simulink model "ADC_Controller_Trajectory_Tracking_Turb"  (R2017b)
settings: Solver=VariableStepAuto  StartTime=0.0  StopTime=200  FixedStep=0.01  RelTol=1e-3
values from neighbouring files (symbols this model uses):
  A_define = A(1:12,1:12)    [F16_init.m]
  A_la_define = A_define([2,4,6,9,10,12],[2,4,6,9,10,12])    [Controller_para.m]
  A_lon_define = A_define([1,3,5,7,8,11],[1,3,5,7,8,11])    [Controller_para.m]
  airSpeed = 393.720000000000    (= 393.72)    [F16_init.m]
  alpha0 = trimAlpha*180/pi    (= 6.62393794015)    [F16_init.m]
  altitude = 9843    [F16_init.m]
  B_define = A(1:12,13:16)    [F16_init.m]
  B_la_define = B_define([2,4,6,9,10,12],3:4)    [Controller_para.m]
  B_lon_define = B_define([1,3,5,7,8,11],1:2)    [Controller_para.m]
  b_ref = 30.0    (= 30)    [F16_init.m]
  C_la = [1,0,zeros(1,4)]    [F16_init.m]
  C_lon = [1,0,zeros(1,4);0,1,zeros(1,4)]    [F16_init.m]
  CC_la = P_la * B_la_define    [Controller_para.m]
  CC_lon = P_lon * B_lon_define    [Controller_para.m]
  dLEF = 0    [F16_init.m]
  fi_flag = 1    [F16_init.m]
  Ki_la = -k_la(:,9)    [F16_init.m]
  Ki_lon = -k_lon(:,9:10)    [F16_init.m]
  kp_la = Kp_define(3:4,[2,4,6,9,10,12])    [Controller_para.m]    (also in F16_init.m)
  kp_lon = Kp_define(1:2,[1,3,5,7,8,11])    [Controller_para.m]    (also in F16_init.m)
  mass = 636.94    [F16_init.m]
  trim_ail = 0.00874607850103852    (= 0.00874607850104)    [F16_init.m]
  trim_control = [trim_thrust;trim_ele;trim_ail;trim_rud]    [F16_init.m]
  trim_ele = -2.97973164860638    (= -2.97973164861)    [F16_init.m]
  trim_rud = 0.0680302158182712    (= 0.0680302158183)    [F16_init.m]
  trim_state = [0;0;0;0;trimAlpha;0;airSpeed;trimAlpha;0;0;0;0]    [F16_init.m]
  trim_thrust = 2279.08519954656    (= 2279.08519955)    [F16_init.m]
undefined symbols (not defined in the file or in its folder): F, MIL
libraries: aerolibconvert2 x7, aerolibasang x4, aerolibobsolete x2, aerolibwind2 x1, aerolibatmos2 x1, aerolibadyn x1
settings Model: Creator=Ma  LastModifiedBy=Jinrui
settings CodeAppCC: StateflowObjectComments=on

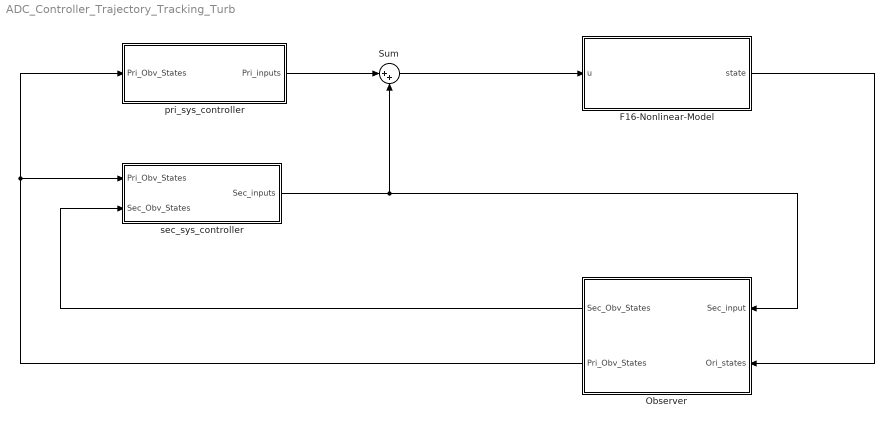
== system ADC_Controller_Trajectory_Tracking_Turb ==
  F16-Nonlinear-Model : Subsystem
  Observer : Subsystem
  Sum : Sum  Inputs=|++
  pri_sys_controller : Subsystem
  sec_sys_controller : Subsystem
  wires:
  pri_sys_controller/1(Pri_inputs) -> Sum/1
  Sum/1 -> F16-Nonlinear-Model/1(u)
  Observer/2(Pri_Obv_States) -> sec_sys_controller/1(Pri_Obv_States), pri_sys_controller/1(Pri_Obv_States)
  Observer/1(Sec_Obv_States) -> sec_sys_controller/2(Sec_Obv_States)
  F16-Nonlinear-Model/1(state) -> Observer/2(Ori_states)
  sec_sys_controller/1(Sec_inputs) -> Sum/2, Observer/1(Sec_input)

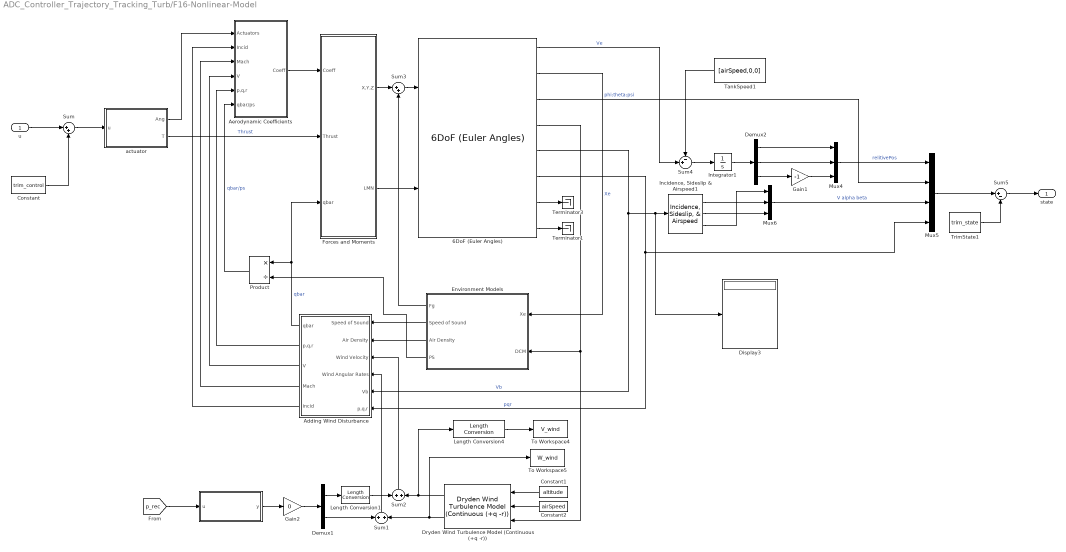
== system ADC_Controller_Trajectory_Tracking_Turb/F16-Nonlinear-Model ==
  u : Inport
  " " : MATLAB Function  TreatAsAtomicUnit=on
  6DoF (Euler Angles) : aerolibobsolete/6DoF (Euler Angles)  units=English (Velocity in ft/s)  mtype=Fixed  rep=Euler Angles  xme_0=xme_0  Vm_0=Vmw  eul_0=Euler_0  pm_0=pm_0  mass_0=mass  mass_e=0.5  mass_f=2.0  inertia=Inertia  inertia_e=eye(3)  inertia_f=2*eye(3)  k_quat=1.0
      settings: SourceProductName=Aerospace Blockset  SourceProductBaseCode=AE
  Adding Wind Disturbance : Subsystem
  Aerodynamic Coefficients : Subsystem
  Constant : Constant  Value=trim_control
  Constant1 : Constant  Value=altitude
  Constant2 : Constant  Value=airSpeed
  Demux1 : Demux  Outputs=2
  Demux2 : Demux  Outputs=3
  Display3 : Display
  Dryden Wind Turbulence Model (Continuous (+q -r)) : aerolibwind2/Dryden Wind Turbulence Model  (Continuous (+q -r))  units=English (Velocity in ft/s)  spec=MIL-F-8785C  model=Continuous Dryden (+q -r)  W20=15  Wdeg=0  TurbProb=10^-1  L_high=533.4  Wingspan=10  ts=0.1  Seed=1+fix(3650*rand(1,4))  T_on=on
      settings: SourceProductName=Aerospace Blockset
  Environment Models : Subsystem
  Forces and Moments : Subsystem
  Gain1 : Gain  Gain=-1
  Gain2 : Gain  Gain=0
  "Incidence, Sideslip & Airspeed1" : aerolibasang/Incidence, Sideslip, & Airspeed
      settings: SourceProductName=Aerospace Blockset
  Integrator1 : Integrator
  Length Conversion1 : aerolibconvert2/Length Conversion  IU=m  OU=ft
  Length Conversion4 : aerolibconvert2/Length Conversion  IU=ft  OU=m
  Mux4 : Mux  Inputs=3
  Mux5 : Mux
  Mux6 : Mux  Inputs=3
  Product : Product  Inputs=*/  SaturateOnIntegerOverflow=on  InputSameDT=on  OutDataTypeStr=Inherit: Same as first input
  Sum : Sum  Inputs=|++
  Sum1 : Sum  Inputs=+|+
  Sum2 : Sum  Inputs=+|+
  Sum3 : Sum  Inputs=|++  SaturateOnIntegerOverflow=on  InputSameDT=on  OutDataTypeStr=Inherit: Same as first input
  Sum4 : Sum  Inputs=-+|
  Sum5 : Sum  Inputs=|+-
  TankSpeed1 : Constant  Value=[airSpeed,0,0]
  Terminator1 : Terminator
  Terminator3 : Terminator
  To Workspace4 : ToWorkspace  VariableName=V_wind  SaveFormat=Structure With Time  SampleTime=-1
  To Workspace5 : ToWorkspace  VariableName=W_wind  SaveFormat=Structure With Time  SampleTime=-1
  TrimState1 : Constant  Value=trim_state
  actuator : Subsystem
  state : Outport
  wires:
  6DoF (Euler Angles)/8 -> Terminator1/1
  6DoF (Euler Angles)/7 -> Terminator3/1
  6DoF (Euler Angles)/4 -> Dryden Wind Turbulence Model (Continuous (+q -r))/3, Environment Models/2(DCM)
  Adding Wind Disturbance/5(Incid) -> Aerodynamic Coefficients/2(Incid)
  Aerodynamic Coefficients/1(Coeff) -> Forces and Moments/1(Coeff)
  Environment Models/2(Speed of Sound) -> Adding Wind Disturbance/1(Speed of Sound)
  Environment Models/3(Air Density) -> Adding Wind Disturbance/2(Air Density)
  Forces and Moments/2(LMN) -> 6DoF (Euler Angles)/2
  Adding Wind Disturbance/1(qbar) -> Forces and Moments/3(qbar), Product/1  "qbar"
  Forces and Moments/1(X,Y,Z) -> Sum3/1
  Sum3/1 -> 6DoF (Euler Angles)/1
  Environment Models/1(Fg) -> Sum3/2
  Adding Wind Disturbance/3(V) -> Aerodynamic Coefficients/4(V)
  Adding Wind Disturbance/4(Mach) -> Aerodynamic Coefficients/3(Mach)
  Adding Wind Disturbance/2("p,q,r ") -> Aerodynamic Coefficients/5(p,q,r)
  Environment Models/4(PS) -> Product/2
  Product/1 -> Aerodynamic Coefficients/6(qbar/ps)  "qbar/ps"
  actuator/2(T) -> Forces and Moments/2(Thrust)  "Thrust"
  actuator/1(Ang) -> Aerodynamic Coefficients/1(Actuators)
  6DoF (Euler Angles)/3 -> Mux5/2  "phi;theta;psi"
  "Incidence, Sideslip & Airspeed1"/1 -> Mux6/2
  "Incidence, Sideslip & Airspeed1"/2 -> Mux6/3
  Mux6/1 -> Mux5/3  "V alpha beta"
  6DoF (Euler Angles)/6 -> Adding Wind Disturbance/6(p,q,r), Mux5/4  "pqr"
  6DoF (Euler Angles)/5 -> Adding Wind Disturbance/5(Vb), Display3/1, "Incidence, Sideslip & Airspeed1"/1  "Vb"
  Mux5/1 -> Sum5/1
  TrimState1/1 -> Sum5/2
  Sum5/1 -> state/1
  Demux2/2 -> Mux4/2
  Demux2/3 -> Gain1/1
  Mux4/1 -> Mux5/1  "relitivePos"
  Demux2/1 -> Mux4/1
  Gain1/1 -> Mux4/3
  Sum4/1 -> Integrator1/1
  Integrator1/1 -> Demux2/1
  6DoF (Euler Angles)/2 -> Environment Models/1(Xe)  "Xe"
  6DoF (Euler Angles)/1 -> Sum4/2  "Ve"
  TankSpeed1/1 -> Sum4/1
  "Incidence, Sideslip & Airspeed1"/3 -> Mux6/1
  Sum/1 -> actuator/1(u)
  Constant/1 -> Sum/2
  u/1 -> Sum/1
  Constant1/1 -> Dryden Wind Turbulence Model (Continuous (+q -r))/1
  Constant2/1 -> Dryden Wind Turbulence Model (Continuous (+q -r))/2
  [p_rec] -> " "/1(u)
  " "/1(y) -> Gain2/1
  Demux1/2 -> Sum1/1
  Sum1/1 -> Adding Wind Disturbance/4(Wind Angular Rates)
  Dryden Wind Turbulence Model (Continuous (+q -r))/1 -> Length Conversion4/1, Sum2/2
  Demux1/1 -> Length Conversion1/1
  Sum2/1 -> Adding Wind Disturbance/3(Wind Velocity)
  Gain2/1 -> Demux1/1
  Length Conversion4/1 -> To Workspace4/1
  Dryden Wind Turbulence Model (Continuous (+q -r))/2 -> To Workspace5/1, Sum1/2
  Length Conversion1/1 -> Sum2/1

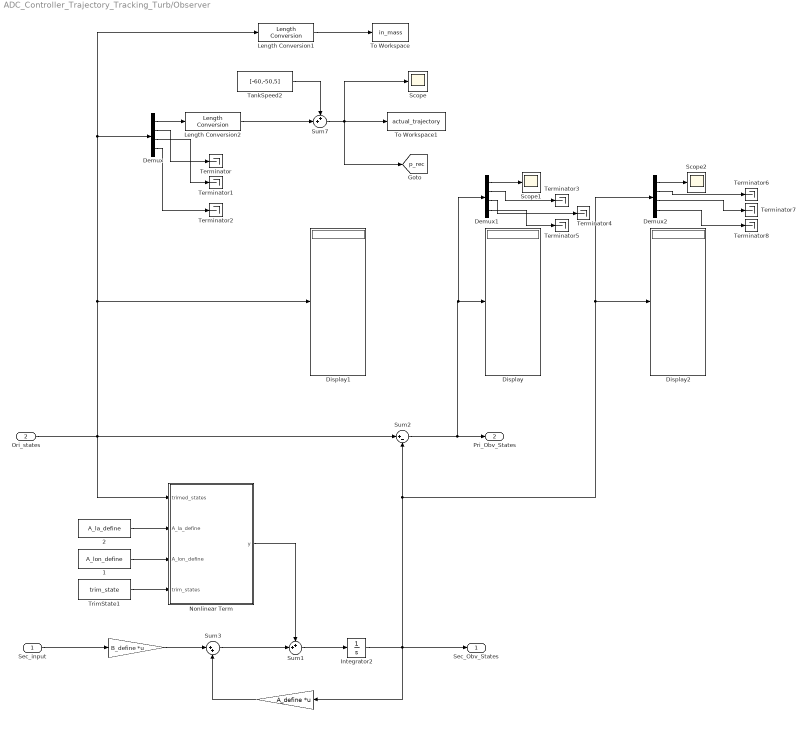
== system ADC_Controller_Trajectory_Tracking_Turb/Observer ==
  Sec_input : Inport
  Ori_states : Inport  Port=2
  " " : Gain  Gain=A_define  Multiplication=Matrix(K*u) (u vector)
  "  " : Gain  Gain=B_define  Multiplication=Matrix(K*u) (u vector)
  " 1" : Constant  Value=A_lon_define
  " 2" : Constant  Value=A_la_define
  Demux : Demux
  Demux1 : Demux
  Demux2 : Demux
  Display : Display
  Display1 : Display
  Display2 : Display
  Integrator2 : Integrator  InitialCondition=zeros(12,1)
  Length Conversion1 : aerolibconvert2/Length Conversion  IU=ft  OU=m
  Length Conversion2 : aerolibconvert2/Length Conversion  IU=ft  OU=m
  Nonlinear Term : MATLAB Function  TreatAsAtomicUnit=on
  Scope : Scope
  Scope1 : Scope
  Scope2 : Scope
  Sum1 : Sum  Inputs=++|
  Sum2 : Sum  Inputs=|+-
  Sum3 : Sum  Inputs=|++
  Sum7 : Sum  Inputs=++|
  TankSpeed2 : Constant  Value=[-60,-50,5]
  Terminator{,1..8} (9 alike) : Terminator
  To Workspace : ToWorkspace  VariableName=in_mass  SaveFormat=Structure With Time  SampleTime=-1
  To Workspace1 : ToWorkspace  VariableName=actual_trajectory  SaveFormat=Structure With Time  SampleTime=-1
  TrimState1 : Constant  Value=trim_state
  Sec_Obv_States : Outport
  Pri_Obv_States : Outport  Port=2
  tag scope: p_rec=global
  wires:
  Sec_input/1 -> "  "/1
  "  "/1 -> Sum3/1
  " "/1 -> Sum3/2
  Sum3/1 -> Sum1/2
  Sum1/1 -> Integrator2/1
  Integrator2/1 -> Sec_Obv_States/1, " "/1, Demux2/1, Display2/1, Sum2/2
  Sum2/1 -> Demux1/1, Display/1, Pri_Obv_States/1
  " 1"/1 -> Nonlinear Term/3(A_lon_define)
  " 2"/1 -> Nonlinear Term/2(A_la_define)
  Demux/1 -> Length Conversion2/1
  Demux1/1 -> Scope1/1
  Demux2/1 -> Scope2/1
  Nonlinear Term/1(y) -> Sum1/1
  TrimState1/1 -> Nonlinear Term/4(trim_states)
  Length Conversion1/1 -> To Workspace/1
  Ori_states/1 -> Sum2/1, Display1/1, Demux/1, Length Conversion1/1, Nonlinear Term/1(trimed_states)
  Length Conversion2/1 -> Sum7/2
  Sum7/1 -> Scope/1, To Workspace1/1, [p_rec]
  TankSpeed2/1 -> Sum7/1
  Demux/2 -> Terminator/1
  Demux/3 -> Terminator1/1
  Demux/4 -> Terminator2/1
  Demux1/2 -> Terminator3/1
  Demux1/3 -> Terminator4/1
  Demux1/4 -> Terminator5/1
  Demux2/4 -> Terminator8/1
  Demux2/3 -> Terminator7/1
  Demux2/2 -> Terminator6/1

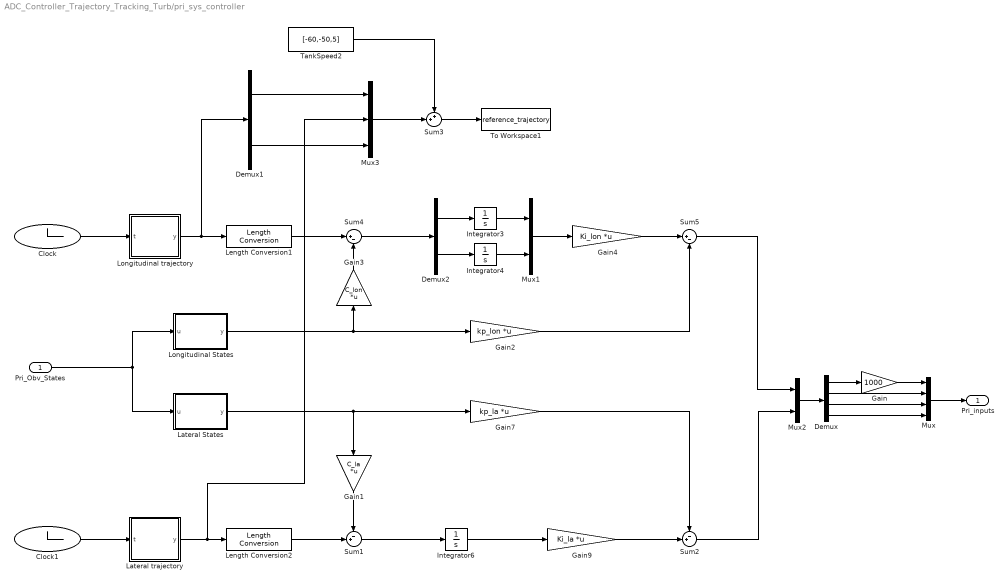
== system ADC_Controller_Trajectory_Tracking_Turb/pri_sys_controller ==
  Pri_Obv_States : Inport
  Clock : Clock
      settings: Decimation=50
  Clock1 : Clock
      settings: Decimation=50
  Demux : Demux
  Demux1 : Demux  Outputs=2
  Demux2 : Demux  Outputs=2
  Gain : Gain  Gain=1000
  Gain1 : Gain  Gain=C_la  Multiplication=Matrix(K*u) (u vector)
  Gain2 : Gain  Gain=kp_lon  Multiplication=Matrix(K*u) (u vector)
  Gain3 : Gain  Gain=C_lon  Multiplication=Matrix(K*u) (u vector)
  Gain4 : Gain  Gain=Ki_lon  Multiplication=Matrix(K*u) (u vector)
  Gain7 : Gain  Gain=kp_la  Multiplication=Matrix(K*u) (u vector)
  Gain9 : Gain  Gain=Ki_la  Multiplication=Matrix(K*u) (u vector)
  Integrator3 : Integrator
  Integrator4 : Integrator
  Integrator6 : Integrator
  Lateral States : MATLAB Function  TreatAsAtomicUnit=on
  Lateral trajectory : MATLAB Function  TreatAsAtomicUnit=on
  Length Conversion1 : aerolibconvert2/Length Conversion  IU=m  OU=ft
  Length Conversion2 : aerolibconvert2/Length Conversion  IU=m  OU=ft
  Longitudinal States : MATLAB Function  TreatAsAtomicUnit=on
  Longitudinal trajectory : MATLAB Function  TreatAsAtomicUnit=on
  Mux : Mux
  Mux1 : Mux  Inputs=2
  Mux2 : Mux  Inputs=2
  Mux3 : Mux  Inputs=3
  Sum1 : Sum  Inputs=-+|
  Sum2 : Sum  Inputs=-+|
  Sum3 : Sum  Inputs=++|
  Sum4 : Sum  Inputs=|+-
  Sum5 : Sum  Inputs=|+-
  TankSpeed2 : Constant  Value=[-60,-50,5]
  To Workspace1 : ToWorkspace  VariableName=reference_trajectory  SaveFormat=Structure With Time  SampleTime=-1
  Pri_inputs : Outport
  wires:
  Pri_Obv_States/1 -> Longitudinal States/1(u), Lateral States/1(u)
  Gain2/1 -> Sum5/2
  Longitudinal trajectory/1(y) -> Demux1/1, Length Conversion1/1
  Sum4/1 -> Demux2/1
  Demux2/2 -> Integrator4/1
  Integrator4/1 -> Mux1/2
  Integrator3/1 -> Mux1/1
  Mux1/1 -> Gain4/1
  Gain3/1 -> Sum4/2
  Gain4/1 -> Sum5/1
  Clock/1 -> Longitudinal trajectory/1(t)
  Length Conversion1/1 -> Sum4/1
  Demux/2 -> Mux/2
  Demux/3 -> Mux/3
  Demux/4 -> Mux/4
  Demux/1 -> Gain/1
  Gain/1 -> Mux/1
  Mux/1 -> Pri_inputs/1
  Lateral trajectory/1(y) -> Mux3/2, Length Conversion2/1
  Sum1/1 -> Integrator6/1
  Integrator6/1 -> Gain9/1
  Clock1/1 -> Lateral trajectory/1(t)
  Longitudinal States/1(y) -> Gain2/1, Gain3/1
  Lateral States/1(y) -> Gain7/1, Gain1/1
  Length Conversion2/1 -> Sum1/2
  Gain1/1 -> Sum1/1
  Gain9/1 -> Sum2/2
  Gain7/1 -> Sum2/1
  Sum5/1 -> Mux2/1
  Sum2/1 -> Mux2/2
  Demux2/1 -> Integrator3/1
  Mux2/1 -> Demux/1
  Demux1/1 -> Mux3/1
  Demux1/2 -> Mux3/3
  Sum3/1 -> To Workspace1/1
  Mux3/1 -> Sum3/2
  TankSpeed2/1 -> Sum3/1

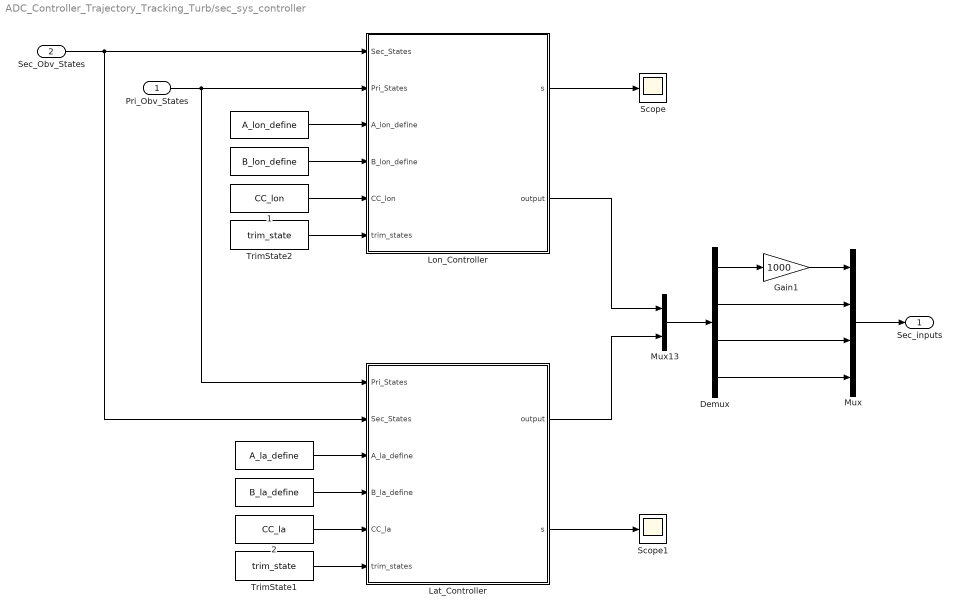
== system ADC_Controller_Trajectory_Tracking_Turb/sec_sys_controller ==
  Pri_Obv_States : Inport
  Sec_Obv_States : Inport  Port=2
  " " : Constant  Value=A_lon_define
  "    " : Constant  Value=B_lon_define
  "     " : Constant  Value=A_la_define
  "      " : Constant  Value=B_la_define
  "    1" : Constant  Value=CC_lon
  "    2" : Constant  Value=CC_la
  Demux : Demux
  Gain1 : Gain  Gain=1000
  Lat_Controller : MATLAB Function  TreatAsAtomicUnit=on
  Lon_Controller : MATLAB Function  TreatAsAtomicUnit=on
  Mux : Mux
  Mux13 : Mux  Inputs=2
  Scope : Scope
  Scope1 : Scope
  TrimState1 : Constant  Value=trim_state
  TrimState2 : Constant  Value=trim_state
  Sec_inputs : Outport
  wires:
  Demux/1 -> Gain1/1
  Gain1/1 -> Mux/1
  Mux/1 -> Sec_inputs/1
  Demux/2 -> Mux/2
  Demux/3 -> Mux/3
  Demux/4 -> Mux/4
  Lon_Controller/2(output) -> Mux13/1
  " "/1 -> Lon_Controller/3(A_lon_define)
  "    "/1 -> Lon_Controller/4(B_lon_define)
  "     "/1 -> Lat_Controller/3(A_la_define)
  "      "/1 -> Lat_Controller/4(B_la_define)
  Lat_Controller/1(output) -> Mux13/2
  "    1"/1 -> Lon_Controller/5(CC_lon)
  "    2"/1 -> Lat_Controller/5(CC_la)
  Lon_Controller/1(s) -> Scope/1
  Lat_Controller/2(s) -> Scope1/1
  Mux13/1 -> Demux/1
  Sec_Obv_States/1 -> Lat_Controller/2(Sec_States), Lon_Controller/1(Sec_States)
  Pri_Obv_States/1 -> Lat_Controller/1(Pri_States), Lon_Controller/2(Pri_States)
  TrimState1/1 -> Lat_Controller/6(trim_states)
  TrimState2/1 -> Lon_Controller/6(trim_states)

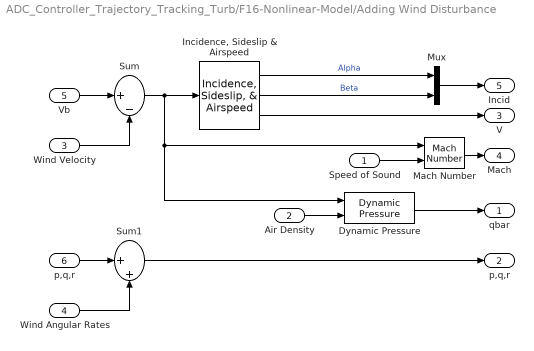
== system ADC_Controller_Trajectory_Tracking_Turb/F16-Nonlinear-Model/Adding Wind Disturbance ==
  Speed of Sound : Inport
  Air Density : Inport  Port=2
  Wind Velocity : Inport  Port=3  PortDimensions=3
  Wind Angular Rates : Inport  Port=4  PortDimensions=3
  Vb : Inport  Port=5  PortDimensions=3
  p,q,r : Inport  Port=6  PortDimensions=3
  Dynamic Pressure : aerolibasang/Dynamic Pressure
  "Incidence, Sideslip & Airspeed" : aerolibasang/Incidence, Sideslip, & Airspeed
      settings: SourceProductName=Aerospace Blockset
  Mach Number : aerolibasang/Mach Number
      settings: SourceProductName=Aerospace Blockset  SourceProductBaseCode=AE
  Mux : Mux  Inputs=2
  Sum : Sum  Inputs=|+-  SaturateOnIntegerOverflow=on  InputSameDT=on  OutDataTypeStr=Inherit: Same as first input
  Sum1 : Sum  Inputs=|++  SaturateOnIntegerOverflow=on  InputSameDT=on  OutDataTypeStr=Inherit: Same as first input
  qbar : Outport  InitialOutput=0
  "p,q,r " : Outport  Port=2
  V : Outport  Port=3
  Mach : Outport  Port=4
  Incid : Outport  Port=5
  wires:
  "Incidence, Sideslip & Airspeed"/3 -> V/1
  Dynamic Pressure/1 -> qbar/1
  Air Density/1 -> Dynamic Pressure/2
  Mach Number/1 -> Mach/1
  Sum/1 -> Dynamic Pressure/1, Mach Number/1, "Incidence, Sideslip & Airspeed"/1
  Vb/1 -> Sum/1
  Speed of Sound/1 -> Mach Number/2
  Wind Velocity/1 -> Sum/2
  "Incidence, Sideslip & Airspeed"/2 -> Mux/2  "Beta"
  Mux/1 -> Incid/1
  "Incidence, Sideslip & Airspeed"/1 -> Mux/1  "Alpha"
  p,q,r/1 -> Sum1/1
  Wind Angular Rates/1 -> Sum1/2
  Sum1/1 -> "p,q,r "/1

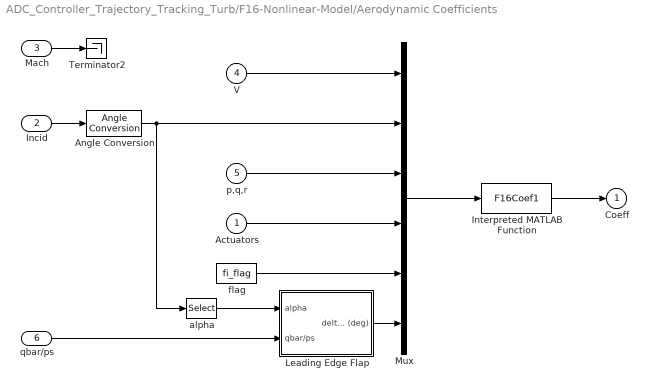
== system ADC_Controller_Trajectory_Tracking_Turb/F16-Nonlinear-Model/Aerodynamic Coefficients ==
  Actuators : Inport
  Incid : Inport  Port=2
  Mach : Inport  Port=3
  V : Inport  Port=4
  p,q,r : Inport  Port=5
  qbar/ps : Inport  Port=6
  Angle Conversion : aerolibconvert2/Angle Conversion  IU=rad  OU=deg
  Interpreted MATLAB Function : MATLABFcn  MATLABFcn=F16Coef1  OutputDimensions=6
  Leading Edge Flap : Subsystem
  Mux : Mux  Inputs=6
  Terminator2 : Terminator
  alpha : Selector  InputPortWidth=2  IndexOptions=Index vector (dialog)  Indices=1  OutputSizes=1
  flag : Constant  Value=fi_flag
  Coeff : Outport  InitialOutput=0
  wires:
  Angle Conversion/1 -> alpha/1, Mux/2
  Incid/1 -> Angle Conversion/1
  qbar/ps/1 -> Leading Edge Flap/2(qbar/ps)
  alpha/1 -> Leading Edge Flap/1(alpha)
  V/1 -> Mux/1
  p,q,r/1 -> Mux/3
  Actuators/1 -> Mux/4
  flag/1 -> Mux/5
  Mach/1 -> Terminator2/1
  Interpreted MATLAB Function/1 -> Coeff/1
  Mux/1 -> Interpreted MATLAB Function/1
  Leading Edge Flap/1(delta_lef (deg)) -> Mux/6

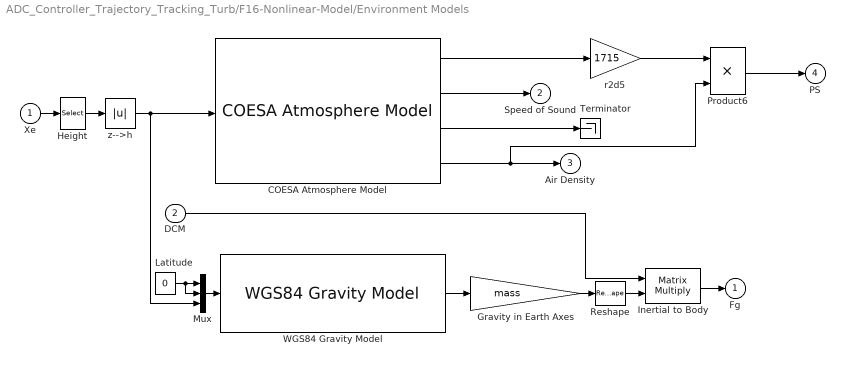
== system ADC_Controller_Trajectory_Tracking_Turb/F16-Nonlinear-Model/Environment Models ==
  Xe : Inport  PortDimensions=3
  DCM : Inport  Port=2
  COESA Atmosphere Model : aerolibatmos2/COESA Atmosphere Model  units=English (Velocity in ft/s)  spec=1976 COESA-extended U.S. Standard Atmosphere  model=Profile  profile_var=High temperature  profile_percent=10%  profile_alt=5 km (16404 ft)  envelope_var=High temperature  envelope_percent=1%  action=None
  Gravity in Earth Axes : Gain  Gain=mass  SaturateOnIntegerOverflow=on  OutDataTypeStr=Inherit: Same as input  ParamDataTypeStr=Inherit: Same as input
  Height : Selector  InputPortWidth=3  IndexOptions=Index vector (dialog)  Indices=[3]  OutputSizes=1
  Inertial to Body : Product  Multiplication=Matrix(*)  SaturateOnIntegerOverflow=on  InputSameDT=on  OutDataTypeStr=Inherit: Same as first input
  Latitude : Constant  Value=0
  Mux : Mux  Inputs=3
  Product6 : Product  Inputs=**  SaturateOnIntegerOverflow=on  InputSameDT=on  OutDataTypeStr=Inherit: Same as first input
  Reshape : Reshape
  Terminator : Terminator
  "WGS84 Gravity Model " : aerolibobsolete/WGS84 Gravity Model   model=WGS84 Taylor Series  units=English  no_atmos=on  precessing=on  jd_loc=off  month=October  day=10  year=2004  no_centrifugal=on  action=None
      settings: SourceProductName=Aerospace Blockset  SourceProductBaseCode=AE
  r2d5 : Gain  Gain=1715  SaturateOnIntegerOverflow=on  OutDataTypeStr=Inherit: Same as input  ParamDataTypeStr=Inherit: Same as input
  z-->h : Abs  SaturateOnIntegerOverflow=on
  Fg : Outport  InitialOutput=0
  Speed of Sound : Outport  Port=2  InitialOutput=0
  Air Density : Outport  Port=3  InitialOutput=0
  PS : Outport  Port=4
  wires:
  Reshape/1 -> Inertial to Body/2
  Mux/1 -> "WGS84 Gravity Model "/1
  z-->h/1 -> Mux/3, COESA Atmosphere Model/1
  COESA Atmosphere Model/2 -> Speed of Sound/1
  COESA Atmosphere Model/3 -> Terminator/1
  Height/1 -> z-->h/1
  Xe/1 -> Height/1
  Latitude/1 -> Mux/2, Mux/1
  "WGS84 Gravity Model "/1 -> Gravity in Earth Axes/1
  Gravity in Earth Axes/1 -> Reshape/1
  DCM/1 -> Inertial to Body/1
  Inertial to Body/1 -> Fg/1
  COESA Atmosphere Model/4 -> Product6/2, Air Density/1
  COESA Atmosphere Model/1 -> r2d5/1
  Product6/1 -> PS/1
  r2d5/1 -> Product6/1

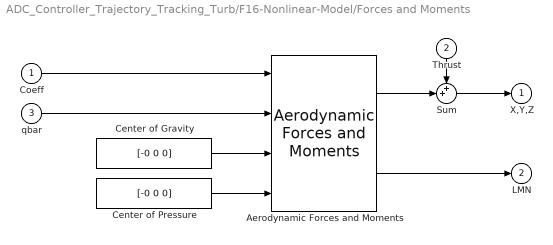
== system ADC_Controller_Trajectory_Tracking_Turb/F16-Nonlinear-Model/Forces and Moments ==
  Coeff : Inport
  Thrust : Inport  Port=2
  qbar : Inport  Port=3
  "Aerodynamic Forces and Moments " : aerolibadyn/Aerodynamic Forces and Moments   inputAxes=Body  outputForceAxes=Body  outputMomentAxes=Body  S=S_ref  b=b_ref  cbar=d_ref
      settings: SourceProductName=Aerospace Blockset
  Center of Gravity : Constant  Value=[-0 0 0]
  Center of Pressure : Constant  Value=[-0 0 0]
  Sum : Sum  Inputs=++|  SaturateOnIntegerOverflow=on  InputSameDT=on  OutDataTypeStr=Inherit: Same as first input
  X,Y,Z : Outport  InitialOutput=0
  LMN : Outport  Port=2  InitialOutput=0
  wires:
  Center of Pressure/1 -> "Aerodynamic Forces and Moments "/4
  Center of Gravity/1 -> "Aerodynamic Forces and Moments "/3
  "Aerodynamic Forces and Moments "/1 -> Sum/2
  "Aerodynamic Forces and Moments "/2 -> LMN/1
  Sum/1 -> X,Y,Z/1
  Thrust/1 -> Sum/1
  qbar/1 -> "Aerodynamic Forces and Moments "/2
  Coeff/1 -> "Aerodynamic Forces and Moments "/1

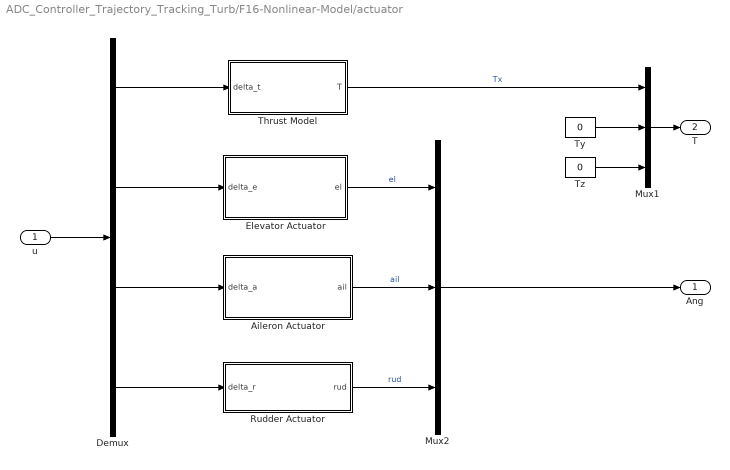
== system ADC_Controller_Trajectory_Tracking_Turb/F16-Nonlinear-Model/actuator ==
  u : Inport
  Aileron Actuator : Subsystem
  Demux : Demux
  Elevator Actuator : Subsystem
  Mux1 : Mux  Inputs=3
  Mux2 : Mux  Inputs=3
  Rudder Actuator : Subsystem
  Thrust Model : Subsystem
  Ty : Constant  Value=0
  Tz : Constant  Value=0
  Ang : Outport
  T : Outport  Port=2
  wires:
  u/1 -> Demux/1
  Mux2/1 -> Ang/1
  Thrust Model/1(T) -> Mux1/1  "Tx"
  Ty/1 -> Mux1/2
  Tz/1 -> Mux1/3
  Mux1/1 -> T/1
  Demux/1 -> Thrust Model/1(delta_t)
  Elevator Actuator/1(el) -> Mux2/1  "el"
  Aileron Actuator/1(ail) -> Mux2/2  "ail"
  Rudder Actuator/1(rud) -> Mux2/3  "rud"
  Demux/2 -> Elevator Actuator/1(delta_e)
  Demux/3 -> Aileron Actuator/1(delta_a)
  Demux/4 -> Rudder Actuator/1(delta_r)

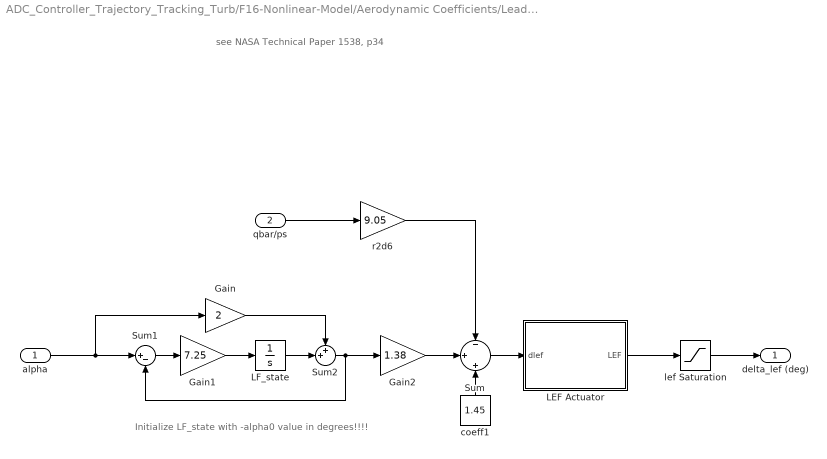
== system ADC_Controller_Trajectory_Tracking_Turb/F16-Nonlinear-Model/Aerodynamic Coefficients/Leading Edge Flap ==
  note: see NASA Technical Paper 1538, p34
  note: Initialize LF_state with -alpha0 value in degrees!!!!
  alpha : Inport
  qbar/ps : Inport  Port=2
  Gain : Gain  Gain=2  SaturateOnIntegerOverflow=on  OutDataTypeStr=Inherit: Same as input  ParamDataTypeStr=Inherit: Same as input
  Gain1 : Gain  Gain=7.25  SaturateOnIntegerOverflow=on  OutDataTypeStr=Inherit: Same as input  ParamDataTypeStr=Inherit: Same as input
  Gain2 : Gain  Gain=1.38  SaturateOnIntegerOverflow=on  OutDataTypeStr=Inherit: Same as input  ParamDataTypeStr=Inherit: Same as input
  LEF Actuator : Subsystem
  LF_state : Integrator  InitialCondition=-alpha0
  Sum : Sum  Inputs=-|+|+  SaturateOnIntegerOverflow=on  InputSameDT=on  OutDataTypeStr=Inherit: Same as first input
  Sum1 : Sum  Inputs=|+-  SaturateOnIntegerOverflow=on  InputSameDT=on  OutDataTypeStr=Inherit: Same as first input
  Sum2 : Sum  Inputs=++|  SaturateOnIntegerOverflow=on  InputSameDT=on  OutDataTypeStr=Inherit: Same as first input
  coeff1 : Constant  Value=1.45
  lef Saturation : Saturate  UpperLimit=25  LowerLimit=0
  r2d6 : Gain  Gain=9.05  SaturateOnIntegerOverflow=on  OutDataTypeStr=Inherit: Same as input  ParamDataTypeStr=Inherit: Same as input
  delta_lef (deg) : Outport
  wires:
  Sum1/1 -> Gain1/1
  Gain1/1 -> LF_state/1
  Gain/1 -> Sum2/1
  Gain2/1 -> Sum/2
  coeff1/1 -> Sum/3
  Sum2/1 -> Sum1/2, Gain2/1
  LF_state/1 -> Sum2/2
  alpha/1 -> Sum1/1, Gain/1
  qbar/ps/1 -> r2d6/1
  r2d6/1 -> Sum/1
  lef Saturation/1 -> delta_lef (deg)/1
  Sum/1 -> LEF Actuator/1(dlef)
  LEF Actuator/1(LEF) -> lef Saturation/1

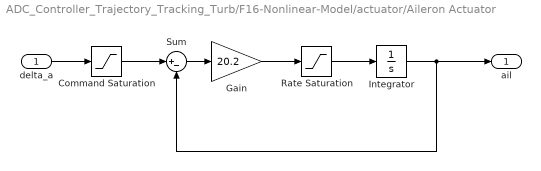
== system ADC_Controller_Trajectory_Tracking_Turb/F16-Nonlinear-Model/actuator/Aileron Actuator ==
  delta_a : Inport
  Command Saturation : Saturate  UpperLimit=21.5  LowerLimit=-21.5
  Gain : Gain  Gain=20.2  SaturateOnIntegerOverflow=on  OutDataTypeStr=Inherit: Same as input  ParamDataTypeStr=Inherit: Same as input
  "Integrator " : Integrator  InitialCondition=trim_ail  UpperSaturationLimit=21.5  LowerSaturationLimit=-21.5
  Rate Saturation : Saturate  UpperLimit=80  LowerLimit=-80
  Sum : Sum  Inputs=|+-  SaturateOnIntegerOverflow=on  InputSameDT=on  OutDataTypeStr=Inherit: Same as first input
  ail : Outport
  wires:
  delta_a/1 -> Command Saturation/1
  "Integrator "/1 -> ail/1, Sum/2
  Sum/1 -> Gain/1
  Gain/1 -> Rate Saturation/1
  Command Saturation/1 -> Sum/1
  Rate Saturation/1 -> "Integrator "/1

== system ADC_Controller_Trajectory_Tracking_Turb/F16-Nonlinear-Model/actuator/Elevator Actuator ==
  delta_e : Inport
  Command Saturation : Saturate  UpperLimit=25  LowerLimit=-25
  Gain : Gain  Gain=20.2  SaturateOnIntegerOverflow=on  OutDataTypeStr=Inherit: Same as input  ParamDataTypeStr=Inherit: Same as input
  "Integrator " : Integrator  InitialCondition=trim_ele  UpperSaturationLimit=25  LowerSaturationLimit=-25
  Rate Saturation : Saturate  UpperLimit=60  LowerLimit=-60
  Sum : Sum  Inputs=|+-  SaturateOnIntegerOverflow=on  InputSameDT=on  OutDataTypeStr=Inherit: Same as first input
  el : Outport
  wires:
  delta_e/1 -> Command Saturation/1
  Command Saturation/1 -> Sum/1
  Sum/1 -> Gain/1
  Gain/1 -> Rate Saturation/1
  "Integrator "/1 -> el/1, Sum/2
  Rate Saturation/1 -> "Integrator "/1

== system ADC_Controller_Trajectory_Tracking_Turb/F16-Nonlinear-Model/actuator/Rudder Actuator ==
  delta_r : Inport
  Command Saturation : Saturate  UpperLimit=30  LowerLimit=-30
  Gain : Gain  Gain=20.2  SaturateOnIntegerOverflow=on  OutDataTypeStr=Inherit: Same as input  ParamDataTypeStr=Inherit: Same as input
  "Integrator " : Integrator  InitialCondition=trim_rud  UpperSaturationLimit=30  LowerSaturationLimit=-30
  Rate Saturation : Saturate  UpperLimit=120  LowerLimit=-120
  Sum : Sum  Inputs=|+-  SaturateOnIntegerOverflow=on  InputSameDT=on  OutDataTypeStr=Inherit: Same as first input
  rud : Outport
  wires:
  "Integrator "/1 -> rud/1, Sum/2
  Sum/1 -> Gain/1
  delta_r/1 -> Command Saturation/1
  Rate Saturation/1 -> "Integrator "/1
  Gain/1 -> Rate Saturation/1
  Command Saturation/1 -> Sum/1

== system ADC_Controller_Trajectory_Tracking_Turb/F16-Nonlinear-Model/actuator/Thrust Model ==
  delta_t : Inport
  Command Saturation : Saturate  UpperLimit=19000  LowerLimit=1000
  Gain : Gain  SaturateOnIntegerOverflow=on  OutDataTypeStr=Inherit: Same as input  ParamDataTypeStr=Inherit: Same as input
  "Integrator " : Integrator  InitialCondition=trim_thrust  UpperSaturationLimit=30  LowerSaturationLimit=-30
  Rate Saturation : Saturate  UpperLimit=10000  LowerLimit=-10000
  Sum : Sum  Inputs=|+-  SaturateOnIntegerOverflow=on  InputSameDT=on  OutDataTypeStr=Inherit: Same as first input
  T : Outport
  wires:
  delta_t/1 -> Command Saturation/1
  Gain/1 -> Rate Saturation/1
  "Integrator "/1 -> T/1, Sum/2
  Command Saturation/1 -> Sum/1
  Sum/1 -> Gain/1
  Rate Saturation/1 -> "Integrator "/1

== system ADC_Controller_Trajectory_Tracking_Turb/F16-Nonlinear-Model/Aerodynamic Coefficients/Leading Edge Flap/LEF Actuator ==
  dlef : Inport
  Command Saturation : Saturate  UpperLimit=25  LowerLimit=0
  Gain3 : Gain  Gain=1/0.136  SaturateOnIntegerOverflow=on  OutDataTypeStr=Inherit: Same as input  ParamDataTypeStr=Inherit: Same as input
  "Integrator " : Integrator  InitialCondition=dLEF  UpperSaturationLimit=21.5  LowerSaturationLimit=-21.5
  Rate Saturation : Saturate  UpperLimit=25  LowerLimit=-25
  Sum3 : Sum  Inputs=|+-  SaturateOnIntegerOverflow=on  InputSameDT=on  OutDataTypeStr=Inherit: Same as first input
  LEF : Outport
  wires:
  Gain3/1 -> Rate Saturation/1
  Rate Saturation/1 -> "Integrator "/1
  "Integrator "/1 -> LEF/1, Sum3/2
  Sum3/1 -> Gain3/1
  dlef/1 -> Command Saturation/1
  Command Saturation/1 -> Sum3/1

== matlab function ADC_Controller_Trajectory_Tracking_Turb/pri_sys_controller/Longitudinal trajectory ==
  settings: updateMethod=DISCRETE
  data: y output; t input
function y = fcn(t)

persistent tt;
if(isempty(tt))
  tt=0;
end

t1 = t-tt;
if t1 < 10
    xx = 0;
elseif  t1 >= 10 && t1 < 70
    xx = 50*sin(0.025*(t1-10));
elseif  t1 >= 70 && t1 < 90
    xx = 50;
elseif  t1 >= 90 && t1 < 150
    xx = 50-15*sin(0.025*(t1-90));
else
    xx = 35;
end

% if t1 < 10
%     xx = 0;
% elseif  t1 >= 10 && t1 < 70
%     xx = 1*sin(0.025*(t1-10));
% else
%     xx = 1;
% end
% xx = 0;

zz = 0;

y = [xx;zz];

end

== matlab function ADC_Controller_Trajectory_Tracking_Turb/F16-Nonlinear-Model/  ==
  data: u input; y output size=6

function y = WindTurFromTank(u)
%#codegen

%横纵向气流角速度等下计算长度
c_lat=4;
c_lon=4;

%两端参考点
u1 = u+[0 ,c_lat ,0]';
u2 = u+[0 ,-c_lat, 0]';

yy1 = TankerVortexWindField(u1);
yy2 = TankerVortexWindField(u2);

%计算x轴向滚转角速度
yp = (yy1(3) - yy2(3))/4/c_lat;

u3=u+[c_lon, 0,0]';
u4=u+[-c_lon ,0,0]';
yy3 = TankerVortexWindField(u3);
yy4 = TankerVortexWindField(u4);

%俯仰角速度计算
yq = -(yy3(3) - yy4(3))/4/c_lon;

%偏航角速度设为0
yr = 0;

%质心处风场计算
y_uvw = TankerVortexWindField(u);

y = [y_uvw(1);y_uvw(2);y_uvw(3);-yp;-yq;-yr];

== matlab function ADC_Controller_Trajectory_Tracking_Turb/sec_sys_controller/Lon_Controller ==
  data: s output; Sec_States input; output output; Pri_States input; A_lon_define input; B_lon_define input; CC_lon input; trim_states input
function [s,output] = Lon_Controller(Sec_States,Pri_States,A_lon_define,B_lon_define,CC_lon,trim_states)
Sec_lon = Sec_States([1,3,5,7,8,11]);  % 辅系统纵向通道状态
ori_states = Sec_States + Pri_States + trim_states;
theta_ori = ori_states(5);
Vr_ori = ori_states(7);
alpha_ori = ori_states(8);

trimed_states = Sec_States + Pri_States;
theta_trimed = trimed_states(5);
Vr_trimed = trimed_states(7);
alpha_trimed = trimed_states(8);

%%  辅系统非线性项g(x)
first_term = Vr_ori * cos(theta_ori - alpha_ori)  - trim_states(7)*cos(trim_states(5)-trim_states(8)) -  A_lon_define(1,3) * theta_trimed - Vr_trimed;
second_term = Vr_ori * sin(theta_ori - alpha_ori) - A_lon_define(2,3) * (theta_trimed - alpha_trimed);
NonLinear = [first_term;second_term;0;0;0;0];
% NonLinear = 0;
%% 滑模控制器结构
s = CC_lon' * Sec_lon;    % 定义滑模面
gain_lon = inv(CC_lon'*B_lon_define);
k1 = [1,0;0,1];
temp = CC_lon'* (A_lon_define * Sec_lon + NonLinear) + k1 * s;
output = -gain_lon * temp;
%% 反馈线性化控制器结构
% s = CC_lon' * Sec_lon;    % 定义输出函数 y = C * x
% gain_lon = inv(CC_lon'*B_lon_define);
% output = gain_lon * (-s - CC_lon' * NonLinear - CC_lon' * A_lon_define * Sec_lon);
end

== matlab function ADC_Controller_Trajectory_Tracking_Turb/sec_sys_controller/Lat_Controller ==
  data: Pri_States input; Sec_States input; output output; A_la_define input; B_la_define input; CC_la input; s output; trim_states input
function [output,s] = Lat_Controller(Pri_States,Sec_States,A_la_define,B_la_define,CC_la,trim_states)
Sec_lat = Sec_States([2,4,6,9,10,12]);  % 辅系统横侧向通道状态
ori_states = Sec_States + Pri_States + trim_states;
phi_ori = ori_states(4);
theta_ori = ori_states(5);
psi_ori = ori_states(6);
Vr_ori = ori_states(7);
alpha_ori = ori_states(8);
beta_ori = ori_states(9);
p_ori = ori_states(10);
q_ori = ori_states(11);
r_ori = ori_states(12);

ug_ori = Vr_ori * cos(alpha_ori) * cos(beta_ori);
vg_ori = Vr_ori * sin(beta_ori);
wg_ori = Vr_ori * sin(alpha_ori) * cos(beta_ori);

yg_ori = ug_ori*cos(theta_ori)*sin(psi_ori) + vg_ori*(sin(phi_ori)*sin(theta_ori)*sin(psi_ori)+cos(phi_ori)*cos(psi_ori)) ...
     + wg_ori*(-sin(phi_ori)*cos(psi_ori)+cos(phi_ori)*sin(theta_ori)*sin(psi_ori));
 
trimed_states = Sec_States + Pri_States;
phi_trimed = trimed_states(4);
theta_trimed = trimed_states(5);
psi_trimed = trimed_states(6);
Vr_trimed = trimed_states(7);
alpha_trimed = trimed_states(8);
beta_trimed = trimed_states(9);
p_trimed = trimed_states(10);
q_trimed = trimed_states(11);
r_trimed = trimed_states(12);
%%  辅系统非线性项g(x)
first_term = yg_ori - A_la_define(1,2) * phi_trimed - A_la_define(1,3) * psi_trimed - A_la_define(1,4) * beta_trimed;
second_term = p_ori + tan(theta_ori)*(q_ori*sin(phi_ori)+r_ori*cos(phi_ori)) - A_la_define(2,5) * p_trimed - A_la_define(2,6) * r_trimed;  % phi
third_term = (q_ori*sin(phi_ori) + r_ori*cos(phi_ori))/cos(theta_ori) - A_la_define(3,6) * r_trimed;  % psi
NonLinear = [first_term;second_term;third_term;0;0;0];
%% 滑模控制器结构
s = CC_la' * Sec_lat;    % 定义滑模面
gain_lat = inv(CC_la'*B_la_define);
k1 = [1,0;0,1];
temp = CC_la'* (A_la_define * Sec_lat + NonLinear) + k1 * s ;
output = -gain_lat * temp;
%% 反馈线性化控制器结构
% s = CC_la' * Sec_lat;    % 定义输出函数 y = C * x
% gain_lat = inv(CC_la'*B_la_define);
% output = gain_lat * (-s - CC_la' * NonLinear - CC_la' * A_la_define * Sec_lat);
end

== matlab function ADC_Controller_Trajectory_Tracking_Turb/pri_sys_controller/Lateral trajectory ==
  settings: updateMethod=DISCRETE
  data: y output; t input
function y = fcn(t)

persistent tt;
if(isempty(tt))
  tt=0;
end

t1 = t-tt;

if t1 < 90
    yy = 0;
elseif  t1 >= 90 && t1 < 150
    yy = 50*sin(0.025*(t1-90));
else
    yy = 50;
end
% end

% yy = 0;
y = yy;

== matlab function ADC_Controller_Trajectory_Tracking_Turb/Observer/Nonlinear Term ==
  data: trimed_states input; y output; A_la_define input; A_lon_define input; trim_states input
function y = fcn(trimed_states,A_la_define,A_lon_define,trim_states)
%% 原状态值（配平前的）
ori_states = trimed_states + trim_states;
phi_ori = ori_states(4);
theta_ori = ori_states(5);
psi_ori = ori_states(6);
Vr_ori = ori_states(7);
alpha_ori = ori_states(8);
beta_ori = ori_states(9);
p_ori = ori_states(10);
q_ori = ori_states(11);
r_ori = ori_states(12);

ug_ori = Vr_ori * cos(alpha_ori) * cos(beta_ori);
vg_ori = Vr_ori * sin(beta_ori);
wg_ori = Vr_ori * sin(alpha_ori) * cos(beta_ori);

xg_ori = ug_ori*cos(theta_ori)*cos(psi_ori) + vg_ori*(sin(phi_ori)*sin(theta_ori)*cos(psi_ori)-cos(phi_ori)*sin(psi_ori)) ...
     + wg_ori*(sin(phi_ori)*sin(psi_ori)+cos(phi_ori)*sin(theta_ori)*cos(psi_ori));
yg_ori = ug_ori*cos(theta_ori)*sin(psi_ori) + vg_ori*(sin(phi_ori)*sin(theta_ori)*sin(psi_ori)+cos(phi_ori)*cos(psi_ori)) ...
     + wg_ori*(-sin(phi_ori)*cos(psi_ori) + cos(phi_ori)*sin(theta_ori)*sin(psi_ori));
hg_ori = ug_ori*sin(theta_ori) - vg_ori*sin(phi_ori)*cos(theta_ori) - wg_ori*cos(phi_ori)*cos(theta_ori);
%% 差状态值（配平后的）
phi_trimed = trimed_states(4);
theta_trimed = trimed_states(5);
psi_trimed = trimed_states(6);
Vr_trimed = trimed_states(7);
alpha_trimed = trimed_states(8);
beta_trimed = trimed_states(9);
p_trimed = trimed_states(10);
q_trimed = trimed_states(11);
r_trimed = trimed_states(12);

% x_nonlinear = Vr_ori * cos(theta_ori - alpha_ori) - A_lon_define(1,3) * theta_trimed - Vr_ori;
% y_nonlinear = Vr_ori * cos(theta_ori - alpha_ori) * sin(psi_ori + beta_ori) - A_la_define(1,2) * phi_trimed - A_la_define(1,3) * psi_trimed - A_la_define(1,4) * beta_trimed;
% h_nonlinear = hg_ori  - A_lon_define(2,3) * (theta_trimed - alpha_trimed);

x_nonlinear = Vr_ori * cos(theta_ori - alpha_ori) - trim_states(7)*cos(trim_states(5)-trim_states(8)) - A_lon_define(1,3) * theta_trimed - Vr_trimed;
y_nonlinear = yg_ori - A_la_define(1,2) * phi_trimed - A_la_define(1,3) * psi_trimed - A_la_define(1,4) * beta_trimed;
h_nonlinear = Vr_ori * sin(theta_ori - alpha_ori) - A_lon_define(2,3) * (theta_trimed - alpha_trimed);
psi_nonlinear = (q_ori*sin(phi_ori) + r_ori*cos(phi_ori))/cos(theta_ori) - A_la_define(3,6) * r_trimed;  % psi
phi_nonlinear = p_ori + tan(theta_ori)*(q_ori*sin(phi_ori)+r_ori*cos(phi_ori)) - A_la_define(2,5) * p_trimed - A_la_define(2,6) * r_trimed;  % phi


y = [x_nonlinear; y_nonlinear; h_nonlinear; phi_nonlinear; 0; psi_nonlinear; 0;0;0;0;0;0];

== matlab function ADC_Controller_Trajectory_Tracking_Turb/pri_sys_controller/Longitudinal States ==
  data: u input; y output
function y = fcn(u)

y = u([1,3,5,7,8,11]);

== matlab function ADC_Controller_Trajectory_Tracking_Turb/pri_sys_controller/Lateral States ==
  data: u input; y output
function y = fcn(u)

y = u([2,4,6,9,10,12]);
